simulink model "conv_AM_system"  (R2021a)
settings: Solver=VariableStepAuto  StartTime=0.0  StopTime=10.0  RelTol=1e-3
settings Model: Creator=Fatiha  LastModifiedBy=Fatiha

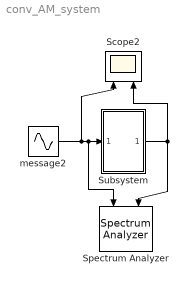
== system conv_AM_system ==
  Scope2 : Scope  NumInputPorts=2
  Spectrum Analyzer : SpectrumAnalyzer  NumInputPorts=2
  Subsystem : Subsystem
  message2 : Sin  Frequency=2*pi*50  Phase=pi/2  SampleTime=0.00001
  wires:
  message2/1 -> Spectrum Analyzer/1, Subsystem/1(In1), Scope2/1
  Subsystem/1(Out1) -> Spectrum Analyzer/2, Scope2/2

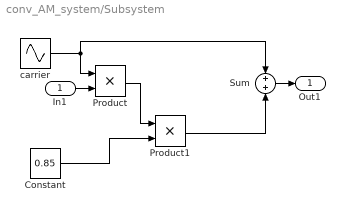
== system conv_AM_system/Subsystem ==
  In1 : Inport
  Constant : Constant  Value=0.85
  Product : Product
  Product1 : Product
  Sum : Sum  Inputs=+|+
  carrier : Sin  Frequency=2*pi*500  Phase=pi/2  SampleTime=0.00001
  Out1 : Outport
  wires:
  Product1/1 -> Sum/2
  In1/1 -> Product/2
  carrier/1 -> Product/1, Sum/1
  Constant/1 -> Product1/2
  Product/1 -> Product1/1
  Sum/1 -> Out1/1
